simulink subsystem "PvtSubSys_VSM_LDW"  (R2020b)
settings: Solver=VariableStepAuto  StartTime=0.0  StopTime=10.0  RelTol=1e-3
values from neighbouring files (symbols this model uses):
  P_VSM_LDW_AbsEspInTime = 3.0    [LDW.sldd]
  P_VSM_LDW_absLongitudeAccIn = 2.5    [LDW.sldd]
  P_VSM_LDW_absLongitudeAccOut = 3.0    [LDW.sldd]
  P_VSM_LDW_AccPedalOut = 30.0    [LDW.sldd]
  P_VSM_LDW_AccRateIn = 30.0    [LDW.sldd]
  P_VSM_LDW_AccRateInTime = 1.5    [LDW.sldd]
  P_VSM_LDW_AccRateOut = 80.0    [LDW.sldd]
  P_VSM_LDW_AccRateOutTime = 0.0    [LDW.sldd]
  P_VSM_LDW_BrakePressIn = 3.0    [LDW.sldd]
  P_VSM_LDW_BrakePressInTime = 1.5    [LDW.sldd]
  P_VSM_LDW_BrakePressOut = 5.0    [LDW.sldd]
  P_VSM_LDW_LaneChangeOffset = 0.11    [LDW.sldd]
  P_VSM_LDW_LaneCurveIn = 0.005    [LDW.sldd]
  P_VSM_LDW_LaneCurveOut = 0.006    [LDW.sldd]
  P_VSM_LDW_LateralAcceIn = 3.0    [LDW.sldd]
  P_VSM_LDW_LateralAcceInTime = 3.0    [LDW.sldd]
  P_VSM_LDW_LateralAcceOut = 3.5    [LDW.sldd]
  P_VSM_LDW_LongitudeAccIn = 3.0    [LDW.sldd]
  P_VSM_LDW_LongitudeAccInTime = 3.0    [LDW.sldd]
  P_VSM_LDW_LongitudeAccOut = 3.5    [LDW.sldd]
  P_VSM_LDW_State_Absesp_enable = 1.0    [LDW.sldd]
  P_VSM_LDW_State_Accpedalrate_enable = 1.0    [LDW.sldd]
  P_VSM_LDW_State_Breakpressure_enable = 1.0    [LDW.sldd]
  P_VSM_LDW_State_ESSSts_enable = 1.0    [LDW.sldd]
  P_VSM_LDW_State_Failsafe_enable = 1.0    [LDW.sldd]
  P_VSM_LDW_State_GEAR_enable = 1.0    [LDW.sldd]
  P_VSM_LDW_State_Headingangle_enable = 1.0    [LDW.sldd]
  P_VSM_LDW_State_Lane_enable = 1.0    [LDW.sldd]
  P_VSM_LDW_State_LaneChange_enable = 1.0    [LDW.sldd]
  P_VSM_LDW_State_Lanecurve_enable = 1.0    [LDW.sldd]
  P_VSM_LDW_State_LateralAcce_enable = 1.0    [LDW.sldd]
  P_VSM_LDW_State_LongitudeAcc_enable = 1.0    [LDW.sldd]
  P_VSM_LDW_State_Param_LaneWidth_Offset : value not decoded    [LDW.sldd]
  P_VSM_LDW_State_Param_REWarningZoneIn = 0.35    [LDW.sldd]
  P_VSM_LDW_State_Param_Sensitive_Offset : value not decoded    [LDW.sldd]
  P_VSM_LDW_State_Param_WarningZoneIn = 0.2    [LDW.sldd]
  P_VSM_LDW_State_Param_WarningZoneOut = -0.65    [LDW.sldd]
  P_VSM_LDW_State_SteerWheelAngle_enable = 1.0    [LDW.sldd]
  P_VSM_LDW_State_SteerWheelSpd_enable = 1.0    [LDW.sldd]
  P_VSM_LDW_State_TurnLight_enable = 1.0    [LDW.sldd]
  P_VSM_LDW_State_Vehspeed_enable = 1.0    [LDW.sldd]
  P_VSM_LDW_State_Yawsup_enable = 1.0    [LDW.sldd]
  P_VSM_LDW_SteerWheelAngleIn = 70.0    [LDW.sldd]
  P_VSM_LDW_SteerWheelAngleInTime = 3.0    [LDW.sldd]
  P_VSM_LDW_SteerWheelAngleOut = 90.0    [LDW.sldd]
  P_VSM_LDW_SteerWheelSpdIn = 150.0    [LDW.sldd]
  P_VSM_LDW_SteerWheelSpdInTime = 3.0    [LDW.sldd]
  P_VSM_LDW_SteerWheelSpdOut = 200.0    [LDW.sldd]
  P_VSM_LDW_TurnLightInTime = 3.0    [LDW.sldd]
  P_VSM_LDW_WhelDy = 2.0    [LDW.sldd]
  P_VSM_LDW_YawRateIn = 0.2    [LDW.sldd]
  P_VSM_LDW_YawRateInTime = 1.0    [LDW.sldd]
  P_VSM_LDW_YawRateOut = 0.25    [LDW.sldd]
undefined symbols (not defined in the file or in its folder): P_VSM_LSMC_SampleTime
libraries: simulink x106
(part 3 of 3)

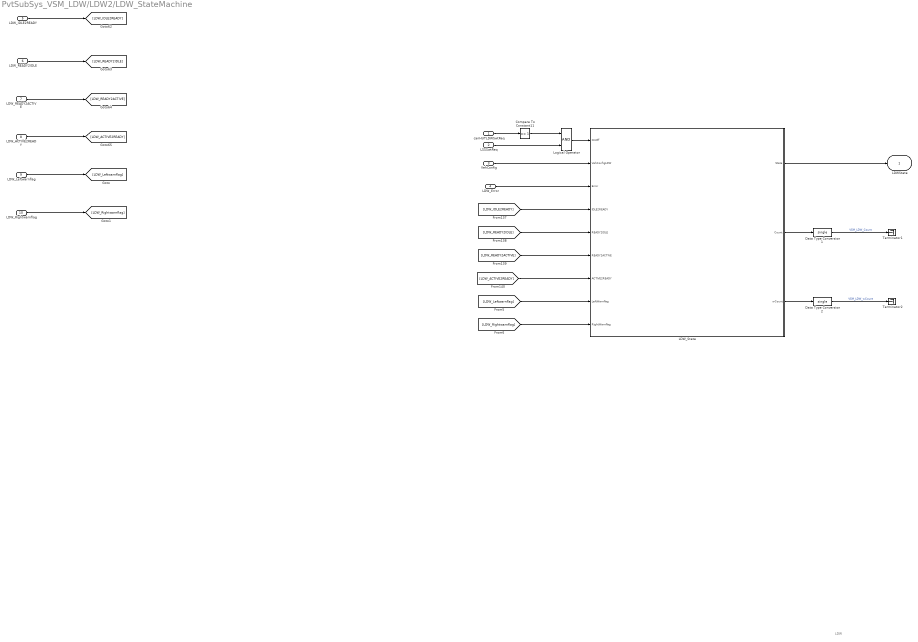
== system PvtSubSys_VSM_LDW/LDW2/LDW_StateMachine ==
  note: LDW
  canHUTLDWSwtReq : Inport
  LSSSwtReq : Inport  Port=2
  VehConfig : Inport  Port=3
  LDW_Error : Inport  Port=4
  LDW_IDLE2READY : Inport  Port=5
  LDW_READY2IDLE : Inport  Port=6
  LDW_READY2ACTIVE : Inport  Port=7
  LDW_ACTIVE2READY : Inport  Port=8
  LDW_Leftwarnflag : Inport  Port=9
  LDW_Rightwarnflag : Inport  Port=10
  Compare To Constant11 : simulink/Logic and Bit Operations/Compare To Constant  relop===  const=1  OutDataTypeStr=boolean
  Data Type Conversion1 : DataTypeConversion  OutDataTypeStr=single
  Data Type Conversion2 : DataTypeConversion  OutDataTypeStr=single
  LDW_State : Stateflow chart  TreatAsAtomicUnit=on
  Logical Operator : Logic  AllPortsSameDT=off  OutDataTypeStr=boolean
  Terminator1 : Terminator
  Terminator2 : Terminator
  LDWState : Outport
  wires:
  [LDW_Rightwarnflag] -> LDW_State/9(RightWarnflag)
  LDW_ACTIVE2READY/1 -> [LDW_ACTIVE2READY]
  LDW_READY2ACTIVE/1 -> [LDW_READY2ACTIVE]
  LDW_READY2IDLE/1 -> [LDW_READY2IDLE]
  LDW_IDLE2READY/1 -> [LDW_IDLE2READY]
  [LDW_ACTIVE2READY] -> LDW_State/7(ACTIVE2READY)
  [LDW_READY2ACTIVE] -> LDW_State/6(READY2ACTIVE)
  LDW_Error/1 -> LDW_State/3(Error)
  canHUTLDWSwtReq/1 -> Compare To Constant11/1
  [LDW_READY2IDLE] -> LDW_State/5(READY2IDLE)
  [LDW_IDLE2READY] -> LDW_State/4(IDLE2READY)
  [LDW_Leftwarnflag] -> LDW_State/8(LeftWarnflag)
  Compare To Constant11/1 -> Logical Operator/1
  LDW_State/2(Count) -> Data Type Conversion1/1
  LDW_State/3(wCount) -> Data Type Conversion2/1
  Data Type Conversion1/1 -> Terminator1/1  "VSM_LDW_Count"
  Data Type Conversion2/1 -> Terminator2/1  "VSM_LDW_wCount"
  LDW_State/1(State) -> LDWState/1
  LDW_Leftwarnflag/1 -> [LDW_Leftwarnflag]
  LDW_Rightwarnflag/1 -> [LDW_Rightwarnflag]
  Logical Operator/1 -> LDW_State/1(OnOff)
  LSSSwtReq/1 -> Logical Operator/2
  VehConfig/1 -> LDW_State/2(VehConfigLDW)

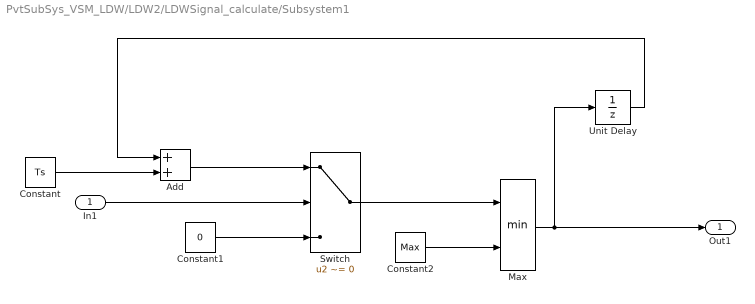
== system PvtSubSys_VSM_LDW/LDW2/LDWSignal_calculate/Subsystem1 ==
  In1 : Inport
  Add : Sum
  Constant : Constant  Value=Ts
  Constant1 : Constant  Value=0
  Constant2 : Constant  Value=Max
  Max : MinMax  Inputs=2
  Switch : Switch  Criteria=u2 ~= 0
  Unit Delay : UnitDelay  SampleTime=-1  HasFrameUpgradeWarning=on
  Out1 : Outport
  wires:
  Unit Delay/1 -> Add/1
  In1/1 -> Switch/2
  Constant/1 -> Add/2
  Constant1/1 -> Switch/3
  Add/1 -> Switch/1
  Max/1 -> Unit Delay/1, Out1/1
  Constant2/1 -> Max/2
  Switch/1 -> Max/1

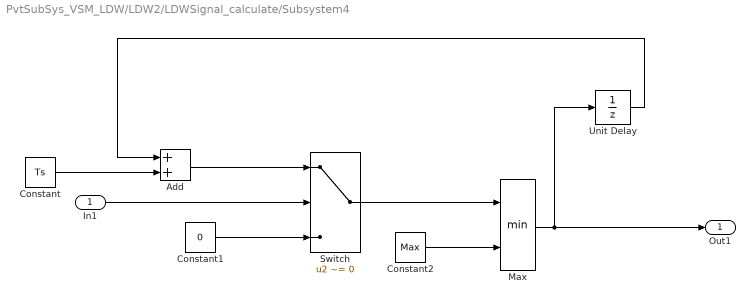
== system PvtSubSys_VSM_LDW/LDW2/LDWSignal_calculate/Subsystem4 ==
  In1 : Inport
  Add : Sum
  Constant : Constant  Value=Ts
  Constant1 : Constant  Value=0
  Constant2 : Constant  Value=Max
  Max : MinMax  Inputs=2
  Switch : Switch  Criteria=u2 ~= 0
  Unit Delay : UnitDelay  SampleTime=-1  HasFrameUpgradeWarning=on
  Out1 : Outport
  wires:
  Switch/1 -> Max/1
  Constant2/1 -> Max/2
  Max/1 -> Out1/1, Unit Delay/1
  Add/1 -> Switch/1
  Constant1/1 -> Switch/3
  Constant/1 -> Add/2
  In1/1 -> Switch/2
  Unit Delay/1 -> Add/1

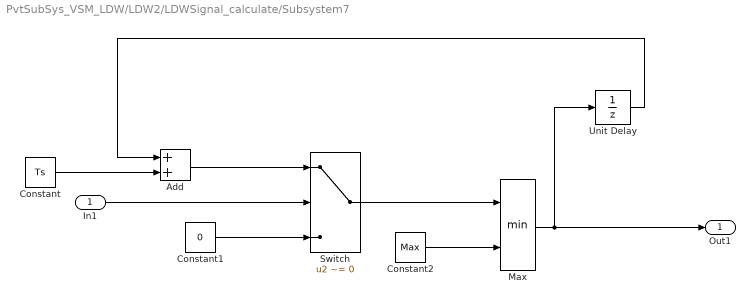
== system PvtSubSys_VSM_LDW/LDW2/LDWSignal_calculate/Subsystem7 ==
  In1 : Inport
  Add : Sum
  Constant : Constant  Value=Ts
  Constant1 : Constant  Value=0
  Constant2 : Constant  Value=Max
  Max : MinMax  Inputs=2
  Switch : Switch  Criteria=u2 ~= 0
  Unit Delay : UnitDelay  SampleTime=-1  HasFrameUpgradeWarning=on
  Out1 : Outport
  wires:
  Unit Delay/1 -> Add/1
  In1/1 -> Switch/2
  Constant/1 -> Add/2
  Constant1/1 -> Switch/3
  Add/1 -> Switch/1
  Max/1 -> Unit Delay/1, Out1/1
  Constant2/1 -> Max/2
  Switch/1 -> Max/1

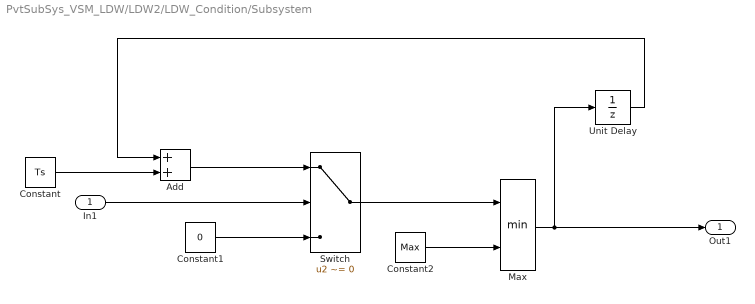
== system PvtSubSys_VSM_LDW/LDW2/LDW_Condition/Subsystem ==
  In1 : Inport
  Add : Sum
  Constant : Constant  Value=Ts
  Constant1 : Constant  Value=0
  Constant2 : Constant  Value=Max
  Max : MinMax  Inputs=2
  Switch : Switch  Criteria=u2 ~= 0
  Unit Delay : UnitDelay  SampleTime=-1  HasFrameUpgradeWarning=on
  Out1 : Outport
  wires:
  Unit Delay/1 -> Add/1
  In1/1 -> Switch/2
  Constant/1 -> Add/2
  Constant1/1 -> Switch/3
  Add/1 -> Switch/1
  Max/1 -> Unit Delay/1, Out1/1
  Constant2/1 -> Max/2
  Switch/1 -> Max/1

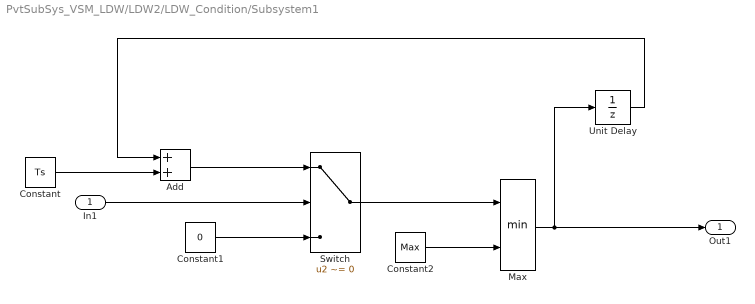
== system PvtSubSys_VSM_LDW/LDW2/LDW_Condition/Subsystem1 ==
  In1 : Inport
  Add : Sum
  Constant : Constant  Value=Ts
  Constant1 : Constant  Value=0
  Constant2 : Constant  Value=Max
  Max : MinMax  Inputs=2
  Switch : Switch  Criteria=u2 ~= 0
  Unit Delay : UnitDelay  SampleTime=-1  HasFrameUpgradeWarning=on
  Out1 : Outport
  wires:
  Unit Delay/1 -> Add/1
  In1/1 -> Switch/2
  Constant/1 -> Add/2
  Constant1/1 -> Switch/3
  Add/1 -> Switch/1
  Max/1 -> Unit Delay/1, Out1/1
  Constant2/1 -> Max/2
  Switch/1 -> Max/1

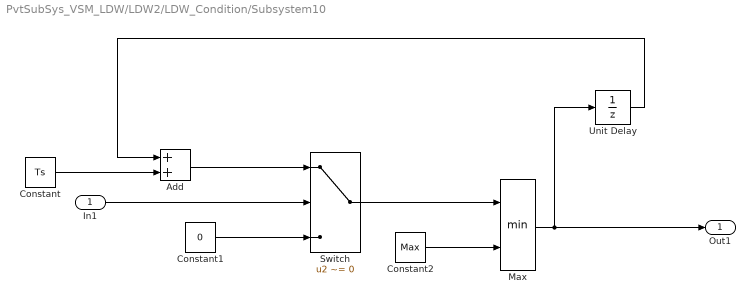
== system PvtSubSys_VSM_LDW/LDW2/LDW_Condition/Subsystem10 ==
  In1 : Inport
  Add : Sum
  Constant : Constant  Value=Ts
  Constant1 : Constant  Value=0
  Constant2 : Constant  Value=Max
  Max : MinMax  Inputs=2
  Switch : Switch  Criteria=u2 ~= 0
  Unit Delay : UnitDelay  SampleTime=-1  HasFrameUpgradeWarning=on
  Out1 : Outport
  wires:
  Switch/1 -> Max/1
  Constant2/1 -> Max/2
  Max/1 -> Out1/1, Unit Delay/1
  Add/1 -> Switch/1
  Constant1/1 -> Switch/3
  Constant/1 -> Add/2
  In1/1 -> Switch/2
  Unit Delay/1 -> Add/1

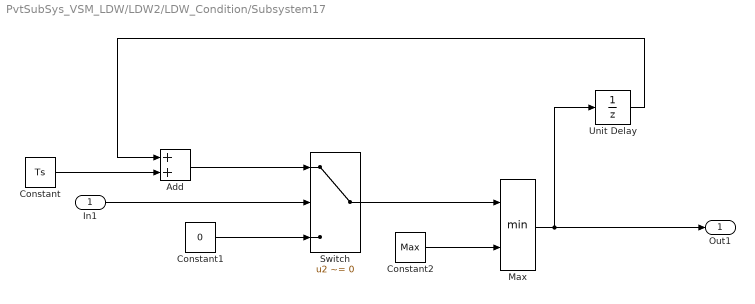
== system PvtSubSys_VSM_LDW/LDW2/LDW_Condition/Subsystem17 ==
  In1 : Inport
  Add : Sum
  Constant : Constant  Value=Ts
  Constant1 : Constant  Value=0
  Constant2 : Constant  Value=Max
  Max : MinMax  Inputs=2
  Switch : Switch  Criteria=u2 ~= 0
  Unit Delay : UnitDelay  SampleTime=-1  HasFrameUpgradeWarning=on
  Out1 : Outport
  wires:
  Switch/1 -> Max/1
  Constant2/1 -> Max/2
  Max/1 -> Out1/1, Unit Delay/1
  Add/1 -> Switch/1
  Constant1/1 -> Switch/3
  Constant/1 -> Add/2
  In1/1 -> Switch/2
  Unit Delay/1 -> Add/1

== system PvtSubSys_VSM_LDW/LDW2/LDW_Condition/Subsystem2 ==
  In1 : Inport
  Add : Sum
  Constant : Constant  Value=Ts
  Constant1 : Constant  Value=0  OutDataTypeStr=single
  Constant2 : Constant  Value=Max  OutDataTypeStr=single
  Max : MinMax  Inputs=2
  Switch : Switch  Criteria=u2 ~= 0
  Unit Delay : UnitDelay  SampleTime=-1  HasFrameUpgradeWarning=on
  Out1 : Outport
  wires:
  Unit Delay/1 -> Add/1
  In1/1 -> Switch/2
  Constant/1 -> Add/2
  Constant1/1 -> Switch/3
  Add/1 -> Switch/1
  Max/1 -> Unit Delay/1, Out1/1
  Constant2/1 -> Max/2
  Switch/1 -> Max/1

== system PvtSubSys_VSM_LDW/LDW2/LDW_Condition/Subsystem3 ==
  In1 : Inport
  Add : Sum
  Constant : Constant  Value=Ts
  Constant1 : Constant  Value=0
  Constant2 : Constant  Value=Max
  Max : MinMax  Inputs=2
  Switch : Switch  Criteria=u2 ~= 0
  Unit Delay : UnitDelay  SampleTime=-1  HasFrameUpgradeWarning=on
  Out1 : Outport
  wires:
  Switch/1 -> Max/1
  Constant2/1 -> Max/2
  Max/1 -> Out1/1, Unit Delay/1
  Add/1 -> Switch/1
  Constant1/1 -> Switch/3
  Constant/1 -> Add/2
  In1/1 -> Switch/2
  Unit Delay/1 -> Add/1

== system PvtSubSys_VSM_LDW/LDW2/LDW_Condition/Subsystem4 ==
  In1 : Inport
  Add : Sum
  Constant : Constant  Value=Ts
  Constant1 : Constant  Value=0
  Constant2 : Constant  Value=Max
  Max : MinMax  Inputs=2
  Switch : Switch  Criteria=u2 ~= 0
  Unit Delay : UnitDelay  SampleTime=-1  HasFrameUpgradeWarning=on
  Out1 : Outport
  wires:
  Unit Delay/1 -> Add/1
  In1/1 -> Switch/2
  Constant/1 -> Add/2
  Constant1/1 -> Switch/3
  Add/1 -> Switch/1
  Max/1 -> Unit Delay/1, Out1/1
  Constant2/1 -> Max/2
  Switch/1 -> Max/1

== system PvtSubSys_VSM_LDW/LDW2/LDW_Condition/Subsystem5 ==
  In1 : Inport
  Add : Sum
  Constant : Constant  Value=Ts
  Constant1 : Constant  Value=0
  Constant2 : Constant  Value=Max
  Max : MinMax  Inputs=2
  Switch : Switch  Criteria=u2 ~= 0
  Unit Delay : UnitDelay  SampleTime=-1  HasFrameUpgradeWarning=on
  Out1 : Outport
  wires:
  Unit Delay/1 -> Add/1
  In1/1 -> Switch/2
  Constant/1 -> Add/2
  Constant1/1 -> Switch/3
  Add/1 -> Switch/1
  Max/1 -> Unit Delay/1, Out1/1
  Constant2/1 -> Max/2
  Switch/1 -> Max/1

== system PvtSubSys_VSM_LDW/LDW2/LDW_Condition/Subsystem6 ==
  In1 : Inport
  Add : Sum
  Constant : Constant  Value=Ts
  Constant1 : Constant  Value=0
  Constant2 : Constant  Value=Max
  Max : MinMax  Inputs=2
  Switch : Switch  Criteria=u2 ~= 0
  Unit Delay : UnitDelay  SampleTime=-1  HasFrameUpgradeWarning=on
  Out1 : Outport
  wires:
  Switch/1 -> Max/1
  Constant2/1 -> Max/2
  Max/1 -> Out1/1, Unit Delay/1
  Add/1 -> Switch/1
  Constant1/1 -> Switch/3
  Constant/1 -> Add/2
  In1/1 -> Switch/2
  Unit Delay/1 -> Add/1

== system PvtSubSys_VSM_LDW/LDW2/LDW_Condition/Subsystem7 ==
  In1 : Inport
  Add : Sum
  Constant : Constant  Value=Ts
  Constant1 : Constant  Value=0
  Constant2 : Constant  Value=Max
  Max : MinMax  Inputs=2
  Switch : Switch  Criteria=u2 ~= 0
  Unit Delay : UnitDelay  SampleTime=-1  HasFrameUpgradeWarning=on
  Out1 : Outport
  wires:
  Unit Delay/1 -> Add/1
  In1/1 -> Switch/2
  Constant/1 -> Add/2
  Constant1/1 -> Switch/3
  Add/1 -> Switch/1
  Max/1 -> Unit Delay/1, Out1/1
  Constant2/1 -> Max/2
  Switch/1 -> Max/1

== system PvtSubSys_VSM_LDW/LDW2/LDW_Condition/Subsystem8 ==
  In1 : Inport
  Add : Sum
  Constant : Constant  Value=Ts
  Constant1 : Constant  Value=0
  Constant2 : Constant  Value=Max
  Max : MinMax  Inputs=2
  Switch : Switch  Criteria=u2 ~= 0
  Unit Delay : UnitDelay  SampleTime=-1  HasFrameUpgradeWarning=on
  Out1 : Outport
  wires:
  Unit Delay/1 -> Add/1
  In1/1 -> Switch/2
  Constant/1 -> Add/2
  Constant1/1 -> Switch/3
  Add/1 -> Switch/1
  Max/1 -> Unit Delay/1, Out1/1
  Constant2/1 -> Max/2
  Switch/1 -> Max/1

== matlab function PvtSubSys_VSM_LDW/LDW2/LDW_Condition/State_TurnLight2 ==
  data: leftlight input; rightlight input; lane input; state output; out output; leftk1 input; left output; rightk1 input; right output
function [state,out,left,right] = fcn(leftlight,rightlight,lane,leftk1,rightk1)
left=0;
right=0;
if leftlight==1 && lane==1  % left alone
    state=1;
    out=0;
    left=1;
elseif lane==1 && leftk1==1  
    state=0;
    out=0;
    left=1;
elseif lane ==1
    state=0;
    out=1;
    left=0;
elseif rightlight==1 && lane==2
    state=1;
    out=0;
    right=1;
elseif lane==2 && rightk1==1
    state=0;
    out=0;
    right=1;
elseif lane ==2
    state=0;
    out=1;
    right=0;
    
else
    state=0;
    out=0;
    left=0;
end

== matlab function PvtSubSys_VSM_LDW/LDW2/LDWSignal_calculate/MATLAB Function1 ==
  data: FLWhelDy input; FRWhelDy input; Left_Valid input; Right_Valid input; LDWLeftwarnflag output single; LDWRightwarnflag output single; ReactionZoneInDy_m input; ReactionZoneOutDy_m input; lfgk1 input; rfgk1 input; lfg output single; rfg output single; loutk1 input; lout output single; routk1 input; rout output single
function [LDWLeftwarnflag,LDWRightwarnflag,lfg,rfg,lout,rout]  = fcn(FLWhelDy,FRWhelDy,Left_Valid,Right_Valid,ReactionZoneInDy_m,ReactionZoneOutDy_m,lfgk1,rfgk1,loutk1,routk1)
LDWLeftwarnflag=single(0);
LDWRightwarnflag=single(0);
lfg=single(0);
rfg=single(0);
lout=single(0);
rout=single(0);
if Left_Valid>single(0)
    if  FLWhelDy<ReactionZoneInDy_m && FLWhelDy>ReactionZoneOutDy_m
        if loutk1==single(1)
            lout=single(1);
            LDWLeftwarnflag=single(0);
            lfg=single(0);
        else
            LDWLeftwarnflag=single(1);
            lfg=single(1);
            lout=single(0);
        end
    elseif FLWhelDy<(ReactionZoneInDy_m+0.1) && FLWhelDy>ReactionZoneOutDy_m && lfgk1>single(0)
        if loutk1==single(1)
            lout=single(1);
            LDWLeftwarnflag=single(0);
            lfg=single(0);
        else
            LDWLeftwarnflag=single(1);
            lfg=single(1);
            lout=single(0);
        end
        
    elseif FLWhelDy < ReactionZoneOutDy_m
        lout=single(1);  
    end
end

if Right_Valid>single(0)
    if  FRWhelDy<ReactionZoneInDy_m && FRWhelDy>ReactionZoneOutDy_m
        if routk1==single(1)
            rout=single(1);
            LDWRightwarnflag=single(0);
            rfg=single(0);
        else
            rout=single(0);
            LDWRightwarnflag=single(1);
            rfg=single(1);
        end
    elseif FRWhelDy<ReactionZoneInDy_m+0.1 &&  FRWhelDy>ReactionZoneOutDy_m  && rfgk1>0
        if routk1==single(1)
            rout=single(1);
            LDWRightwarnflag=single(0);
            rfg=single(0);
        else
            rout=single(0);
            LDWRightwarnflag=single(1);
            rfg=single(1);
        end
        
    elseif FRWhelDy < ReactionZoneOutDy_m
        rout=single(1);
    end
end

== matlab function PvtSubSys_VSM_LDW/LDW2/LDW_Condition/MATLAB Function ==
  data: LeftChangefg input; y output; RightChangefg input; Ldy input; Rdy input; Lfgk1 input; Lfg output; Rfgk1 input; Rfg output
function [y,Lfg,Rfg] = fcn(LeftChangefg,RightChangefg,Ldy,Rdy,Lfgk1,Rfgk1)
y=1;
Lfg=0;
Rfg=0;
if LeftChangefg>0
    Lfg=1;
    y=0;
elseif Lfgk1>0
    Lfg=1;
    y=0;
    if Rdy>0
        Lfg=0;
        y=1;
    end
    
end

if RightChangefg>0
    Rfg=1;
    y=0;
elseif Rfgk1>0
    Rfg=1;
    y=0;
    if Ldy>0
        Rfg=0;
        y=1;
    end
    
end

== stateflow chart PvtSubSys_VSM_LDW/LDW2/LDW_StateMachine/LDW_State ==
  state MAINST_OFF
    entry: State=STATE.OFF;
  state MAINST_ERROR
    entry: State=STATE.ERROR;
  state MAINST_ON
    state SUBST_IDLE
      entry: State=STATE.IDLE;
    state inactive
      state SUBST_READY
        entry: State=STATE.READY;wCount=0;
      state SUBST_ACTIVE
        state LEFT_WARN
          entry: State=STATE.ACTIVE_LEFT;Count=0;
          du:wCount = wCount + 1;
        state RIGHT_WARN
          entry: State=STATE.ACTIVE_RIGHT;Count=0;
          du:wCount = wCount + 1;
        state TIMEOUT
          en:State=STATE.DEFAULT;wCount=0;
          du:Count = Count + 1;
        (junction 25) -> LEFT_WARN [order 1] : [LeftWarnflag==1]
        (junction 25) -> RIGHT_WARN [order 2] : [RightWarnflag==1]
        TIMEOUT -> (junction 25) : [Count>149]{Count=0;}
        LEFT_WARN -> TIMEOUT : [wCount>199]
        RIGHT_WARN -> TIMEOUT : [wCount>199]
      (default) -> SUBST_READY
      SUBST_READY -> (junction 25) : [READY2ACTIVE&&(LeftWarnflag>0||RightWarnflag>0)]
      SUBST_ACTIVE -> SUBST_READY : [ACTIVE2READY||(LeftWarnflag==0&&RightWarnflag==0)]
    (default) -> SUBST_IDLE
    SUBST_IDLE -> inactive : [IDLE2READY && LeftWarnflag==0 && RightWarnflag==0 && Error~=3]
    inactive -> SUBST_IDLE : [READY2IDLE || Error==3]
  (default) -> MAINST_OFF
  MAINST_ERROR -> MAINST_OFF [order 2] : [OnOff==false]
  MAINST_OFF -> MAINST_ON : [OnOff==true  && VehConfigLDW==1]
  MAINST_ON -> MAINST_OFF [order 2] : [OnOff==false]
  MAINST_ON -> MAINST_ERROR [order 1] : [Error== 1 ]
  MAINST_ERROR -> MAINST_ON [order 1] : [Error~=1]
  data: OnOff input; VehConfigLDW input uint8; Error input; IDLE2READY input; READY2IDLE input; READY2ACTIVE input; ACTIVE2READY input; LeftWarnflag input; State output Enum: STATE =STATE.OFF; Count output =0; wCount output =0; RightWarnflag input
